simulink model "multilevelinverterc"  (R2014b)
settings: Solver=ode45  StartTime=0.0  StopTime=0.1  MaxStep=.00001  RelTol=1e-3
libraries: powerlib x58, simulink x10
settings Model: Creator=Muruganandham  LastModifiedBy=SELVA
settings DataIOCC: SignalLoggingSaveFormat=ModelDataLogs
settings OptimizationCC: ExpressionDepthLimit=2147483647
settings DebuggingCC: UnderspecifiedInitializationDetection=Classic  MergeDetectMultiDrivingBlocksExec=none  FcnCallInpInsideContextMsg=UseLocalSettings  StateNameClashWarn=warning
settings GRTTargetCC: CombineOutputUpdateFcns=off  GRTInterface=on

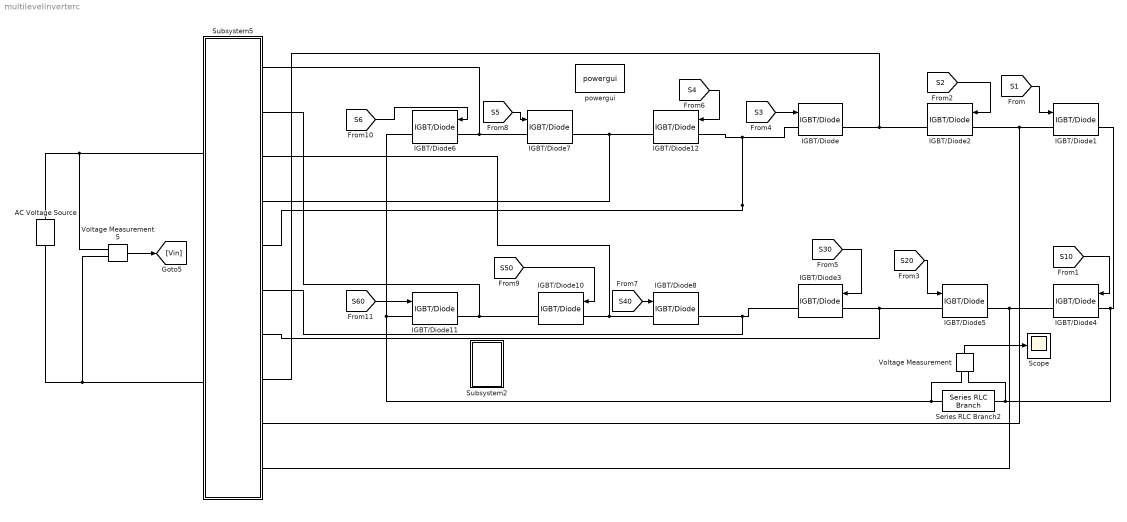
== system multilevelinverterc ==
  AC Voltage Source : powerlib/Electrical Sources/AC Voltage Source  Amplitude=230*sqrt(2)  Phase=0  Frequency=50  SampleTime=0  Measurements=None
  IGBT/Diode{,1..8,10..12} (12 alike) : powerlib/Power Electronics/IGBT//Diode  Ron=1e-3  Rs=1e5  Cs=inf  Measurements=on
  Scope : Scope
      settings: YMin=-600  YMax=600  SaveName=bh
  Series RLC Branch2 : powerlib/Elements/Series RLC Branch  LConnTagsString=__new0  RConnTagsString=__new0  BranchType=R  Resistance=10  Inductance=1e-3  SetiL0=off  InitialCurrent=0  Capacitance=1e-6  Setx0=off  InitialVoltage=0  Measurements=None
  Subsystem2 : Subsystem  mask{fc=10000, m=1}
      mask prompts: fc "Switching frequency"; m "modulation index"
  Subsystem5 : Subsystem
  Voltage Measurement : powerlib/Measurements/Voltage Measurement  PhasorSimulation=off  OutputType=Complex  PSBequivalent=0
  Voltage Measurement5 : powerlib/Measurements/Voltage Measurement  PhasorSimulation=off  OutputType=Complex  PSBequivalent=0
  powergui : powerlib/powergui  Priority=1  SimulationMode=Discrete  SolverType=Tustin  SampleTime=50e-6  frequency=60  SPID=off  DisableSnubberDevices=off  DisableRonSwitches=off  DisableVfSwitches=off  SwTol=0  DisplayEquations=off  Interpol=off  methode=off  Ts=0  frequencyindice=0  Pbase=100e6  ErrMax=1e-4  Iterations=50  UnitsV=kV  UnitsW=MW  FunctionMessages=off  echomessages=off  HookPort=off  EnableUseOfTLC=off  x0status=blocks  RestoreLinks=warning  ResistiveCurrentMeasurement=off  Frange=[0:2:500]  Ylog=off  Xlog=on  ShowGrid=off  save=off  variable=ZData  structure=bh  ZoomFFT=off  StartTime=0.04  cycles=1  DisplayStyle=1  fundamental=50  FreqAxis=off  MaxFrequency=10000  frequencyindicesteady=1  RmsSteady=1  display=off
  wires:
  [S1] -> IGBT/Diode1/1
  [S10] -> IGBT/Diode4/1
  [S2] -> IGBT/Diode2/1
  [S20] -> IGBT/Diode5/1
  [S3] -> IGBT/Diode/1
  [S30] -> IGBT/Diode3/1
  Voltage Measurement/1 -> Scope/1
  [S40] -> IGBT/Diode8/1
  [S6] -> IGBT/Diode6/1
  [S4] -> IGBT/Diode12/1
  [S5] -> IGBT/Diode7/1
  [S50] -> IGBT/Diode10/1
  [S60] -> IGBT/Diode11/1
  Voltage Measurement5/1 -> [Vin]
  connections:
  IGBT/Diode/RConn1 -- Subsystem5/RConn8 -- IGBT/Diode2/RConn1
  IGBT/Diode1/LConn1 -- IGBT/Diode2/LConn1 -- Subsystem5/RConn9
  IGBT/Diode3/LConn1 -- Subsystem5/RConn7 -- IGBT/Diode5/LConn1
  IGBT/Diode5/RConn1 -- Subsystem5/RConn10 -- IGBT/Diode4/RConn1
  IGBT/Diode1/RConn1 -- Voltage Measurement/LConn2 -- Series RLC Branch2/RConn1 -- IGBT/Diode4/LConn1
  IGBT/Diode6/LConn1 -- Subsystem5/RConn1 -- IGBT/Diode7/LConn1
  IGBT/Diode7/RConn1 -- Subsystem5/RConn4 -- IGBT/Diode12/RConn1
  IGBT/Diode11/RConn1 -- Subsystem5/RConn2 -- IGBT/Diode10/RConn1
  IGBT/Diode10/LConn1 -- Subsystem5/RConn3 -- IGBT/Diode8/LConn1
  IGBT/Diode/LConn1 -- Subsystem5/RConn5 -- IGBT/Diode12/LConn1
  IGBT/Diode3/RConn1 -- Subsystem5/RConn6 -- IGBT/Diode8/RConn1
  Series RLC Branch2/LConn1 -- IGBT/Diode11/LConn1 -- IGBT/Diode6/RConn1 -- Voltage Measurement/LConn1
  Voltage Measurement5/LConn1 -- AC Voltage Source/RConn1 -- Subsystem5/LConn1
  Voltage Measurement5/LConn2 -- AC Voltage Source/LConn1 -- Subsystem5/LConn2

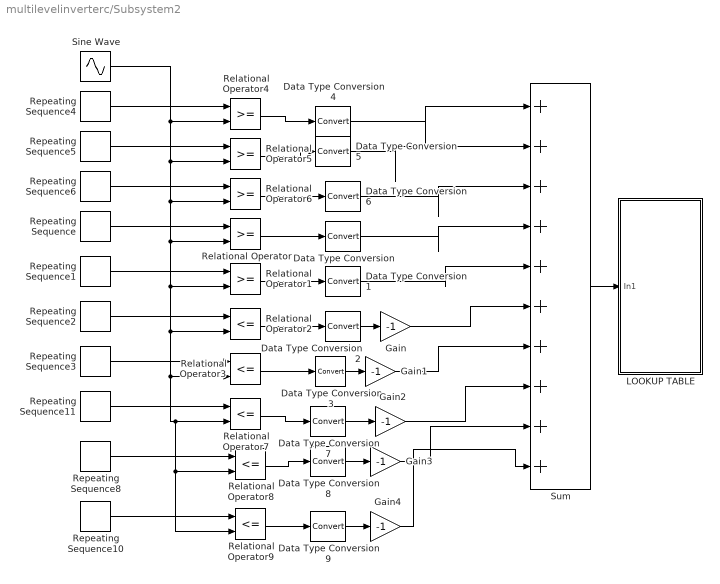
== system multilevelinverterc/Subsystem2 ==
  Data Type Conversion{,1..9} (10 alike) : DataTypeConversion
  Gain{,1..4} (5 alike) : Gain  Gain=-1
  LOOKUP TABLE : Subsystem
  Relational Operator{,1,4..6} (5 alike) : RelationalOperator  OutDataTypeStr=boolean
  Relational Operator{2..3,7..9} (5 alike) : RelationalOperator  Operator=<=  OutDataTypeStr=boolean
  Repeating Sequence : simulink/Sources/Repeating Sequence  rep_seq_t="[0 (1/fc)/2  (1/fc)]"  rep_seq_y=[2 1 2]
  Repeating Sequence1 : simulink/Sources/Repeating Sequence  rep_seq_t="[0 (1/fc)/2  (1/fc)]"  rep_seq_y=[1 0 1]
  Repeating Sequence10 : simulink/Sources/Repeating Sequence  rep_seq_t="[0 (1/fc)/2  (1/fc)]"  rep_seq_y=[-5 -4 -5]
  Repeating Sequence11 : simulink/Sources/Repeating Sequence  rep_seq_t="[0 (1/fc)/2  (1/fc)]"  rep_seq_y=[-3 -2 -3]
  Repeating Sequence2 : simulink/Sources/Repeating Sequence  rep_seq_t="[0 (1/fc)/2  (1/fc)]"  rep_seq_y=[-1 0 -1]
  Repeating Sequence3 : simulink/Sources/Repeating Sequence  rep_seq_t="[0 (1/fc)/2  (1/fc)]"  rep_seq_y=[-2 -1 -2]
  Repeating Sequence4 : simulink/Sources/Repeating Sequence  rep_seq_t="[0 (1/fc)/2  (1/fc)]"  rep_seq_y=[4 5 4]
  Repeating Sequence5 : simulink/Sources/Repeating Sequence  rep_seq_t="[0 (1/fc)/2  (1/fc)]"  rep_seq_y=[4 3 4]
  Repeating Sequence6 : simulink/Sources/Repeating Sequence  rep_seq_t="[0 (1/fc)/2  (1/fc)]"  rep_seq_y=[3 2 3]
  Repeating Sequence8 : simulink/Sources/Repeating Sequence  rep_seq_t="[0 (1/fc)/2  (1/fc)]"  rep_seq_y=[-4 -3 -4]
  Sine Wave : Sin  Amplitude=5*m  Frequency=2*pi*50  SampleTime=0
  Sum : Sum  Inputs=|++++++++++
  wires:
  Data Type Conversion3/1 -> Gain1/1
  Data Type Conversion2/1 -> Gain/1
  Relational Operator3/1 -> Data Type Conversion3/1
  Relational Operator2/1 -> Data Type Conversion2/1
  Repeating Sequence3/1 -> Relational Operator3/1
  Repeating Sequence2/1 -> Relational Operator2/1
  Repeating Sequence1/1 -> Relational Operator1/1
  Repeating Sequence/1 -> Relational Operator/1
  Relational Operator1/1 -> Data Type Conversion1/1
  Relational Operator/1 -> Data Type Conversion/1
  Repeating Sequence6/1 -> Relational Operator6/1
  Repeating Sequence5/1 -> Relational Operator5/1
  Repeating Sequence4/1 -> Relational Operator4/1
  Relational Operator6/1 -> Data Type Conversion6/1
  Relational Operator5/1 -> Data Type Conversion5/1
  Relational Operator4/1 -> Data Type Conversion4/1
  Repeating Sequence8/1 -> Relational Operator8/1
  Repeating Sequence11/1 -> Relational Operator7/1
  Relational Operator9/1 -> Data Type Conversion9/1
  Relational Operator8/1 -> Data Type Conversion8/1
  Relational Operator7/1 -> Data Type Conversion7/1
  Data Type Conversion9/1 -> Gain4/1
  Data Type Conversion8/1 -> Gain3/1
  Data Type Conversion7/1 -> Gain2/1
  Repeating Sequence10/1 -> Relational Operator9/1
  Data Type Conversion4/1 -> Sum/1
  Data Type Conversion5/1 -> Sum/2
  Data Type Conversion6/1 -> Sum/3
  Data Type Conversion/1 -> Sum/4
  Data Type Conversion1/1 -> Sum/5
  Gain/1 -> Sum/6
  Gain1/1 -> Sum/7
  Gain2/1 -> Sum/8
  Gain3/1 -> Sum/9
  Gain4/1 -> Sum/10
  Sum/1 -> LOOKUP TABLE/1(In1)
  Sine Wave/1 -> Relational Operator5/2, Relational Operator6/2, Relational Operator/2, Relational Operator1/2, Relational Operator2/2, Relational Operator3/2, Relational Operator7/2, Relational Operator9/2, Relational Operator8/2, Relational Operator4/2

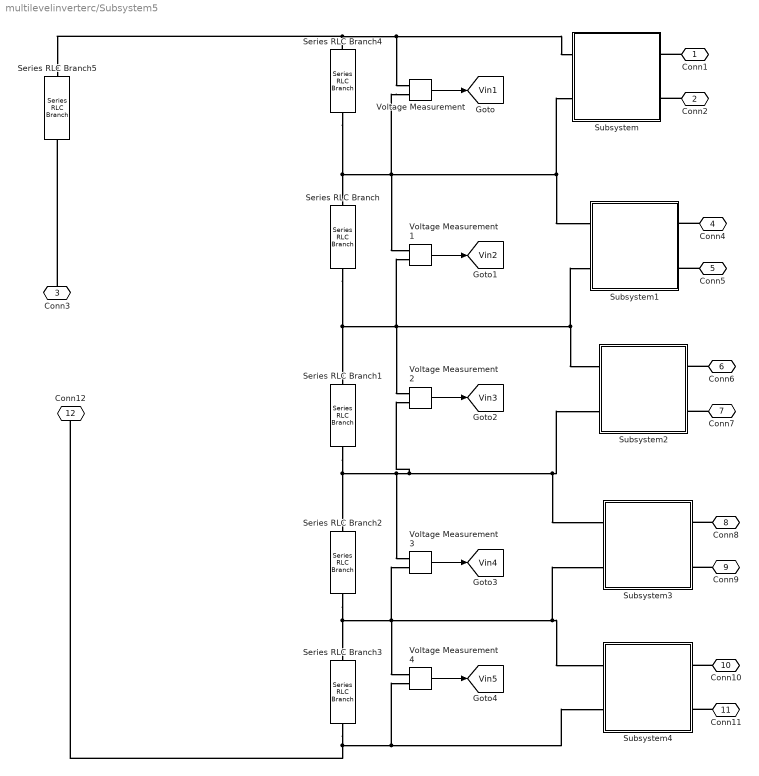
== system multilevelinverterc/Subsystem5 ==
  Series RLC Branch{,1..4} (5 alike) : powerlib/Elements/Series RLC Branch  LConnTagsString=__new0  RConnTagsString=__new0  BranchType=C  Resistance=1  Inductance=1e-3  SetiL0=off  InitialCurrent=0  Capacitance=2500e-6  Setx0=off  InitialVoltage=0  Measurements=None
  Series RLC Branch5 : powerlib/Elements/Series RLC Branch  LConnTagsString=__new0  RConnTagsString=__new0  BranchType=R  Resistance=.001  Inductance=1e-3  SetiL0=off  InitialCurrent=0  Capacitance=2500e-6  Setx0=off  InitialVoltage=0  Measurements=None
  Subsystem : Subsystem
  Subsystem1 : Subsystem
  Subsystem2 : Subsystem
  Subsystem3 : Subsystem
  Subsystem4 : Subsystem
  Voltage Measurement{,1..4} (5 alike) : powerlib/Measurements/Voltage Measurement  PhasorSimulation=off  OutputType=Complex  PSBequivalent=0
  Conn1 : PMIOPort  Port=1  Side=Right
  Conn2 : PMIOPort  Port=2  Side=Right
  Conn3 : PMIOPort  Port=3  Side=Left
  Conn4 : PMIOPort  Port=4  Side=Right
  Conn5 : PMIOPort  Port=5  Side=Right
  Conn6 : PMIOPort  Port=6  Side=Right
  Conn7 : PMIOPort  Port=7  Side=Right
  Conn8 : PMIOPort  Port=8  Side=Right
  Conn9 : PMIOPort  Port=9  Side=Right
  Conn10 : PMIOPort  Port=10  Side=Right
  Conn11 : PMIOPort  Port=11  Side=Right
  Conn12 : PMIOPort  Port=12  Side=Left
  tag scope: Vin1=global, Vin2=global, Vin3=global, Vin4=global, Vin5=global
  wires:
  Voltage Measurement/1 -> [Vin1]
  Voltage Measurement1/1 -> [Vin2]
  Voltage Measurement2/1 -> [Vin3]
  Voltage Measurement3/1 -> [Vin4]
  Voltage Measurement4/1 -> [Vin5]
  connections:
  Voltage Measurement/LConn2 -- Series RLC Branch4/RConn1 -- Series RLC Branch/LConn1 -- Subsystem/LConn2 -- Subsystem1/LConn1 -- Voltage Measurement1/LConn1
  Voltage Measurement1/LConn2 -- Series RLC Branch/RConn1 -- Series RLC Branch1/LConn1 -- Subsystem1/LConn2 -- Subsystem2/LConn1 -- Voltage Measurement2/LConn1
  Series RLC Branch1/RConn1 -- Subsystem2/LConn2 -- Subsystem3/LConn1 -- Voltage Measurement2/LConn2 -- Voltage Measurement3/LConn1 -- Series RLC Branch2/LConn1
  Series RLC Branch2/RConn1 -- Series RLC Branch3/LConn1 -- Subsystem3/LConn2 -- Subsystem4/LConn1 -- Voltage Measurement3/LConn2 -- Voltage Measurement4/LConn1
  Series RLC Branch3/RConn1 -- Conn12/RConn1 -- Subsystem4/LConn2 -- Voltage Measurement4/LConn2
  Series RLC Branch4/LConn1 -- Subsystem/LConn1 -- Voltage Measurement/LConn1 -- Series RLC Branch5/LConn1
  Conn1/RConn1 -- Subsystem/RConn1
  Conn2/RConn1 -- Subsystem/RConn2
  Conn3/RConn1 -- Series RLC Branch5/RConn1
  Conn4/RConn1 -- Subsystem1/RConn1
  Conn5/RConn1 -- Subsystem1/RConn2
  Conn6/RConn1 -- Subsystem2/RConn1
  Conn7/RConn1 -- Subsystem2/RConn2
  Conn8/RConn1 -- Subsystem3/RConn1
  Conn9/RConn1 -- Subsystem3/RConn2
  Conn10/RConn1 -- Subsystem4/RConn1
  Conn11/RConn1 -- Subsystem4/RConn2

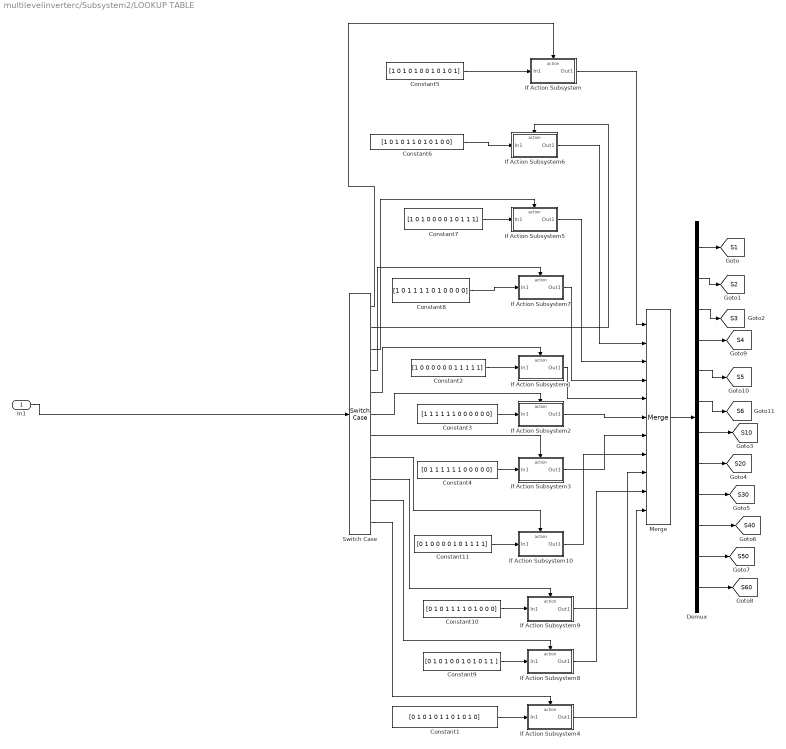
== system multilevelinverterc/Subsystem2/LOOKUP TABLE ==
  In1 : Inport
  Constant1 : Constant  Value=[0 1 0 1 0 1 1 0 1 0 1 0]
  Constant10 : Constant  Value=[0 1 0 1 1 1 1 0 1 0 0 0]
  Constant11 : Constant  Value=[0 1 0 0 0 0 1 0 1 1 1 1]
  Constant2 : Constant  Value=[1 0 0 0 0 0 0 1 1 1 1 1]
  Constant3 : Constant  Value=[1 1 1 1 1 1 0 0 0 0 0 0]
  Constant4 : Constant  Value=[0 1 1 1 1 1 1 0 0 0 0 0]
  Constant5 : Constant  Value=[1 0 1 0 1 0 0 1 0 1 0 1]
  Constant6 : Constant  Value=[1 0 1 0 1 1 0 1 0 1 0 0]
  Constant7 : Constant  Value=[1 0 1 0 0 0 0 1 0 1 1 1]
  Constant8 : Constant  Value=[1 0 1 1 1 1 0 1 0 0 0 0]
  Constant9 : Constant  Value=[0 1 0 1 0 0 1 0 1 0 1 1 ]
  Demux : Demux  Outputs=12
  If Action Subsystem : Subsystem  TreatAsAtomicUnit=on
  If Action Subsystem1 : Subsystem  TreatAsAtomicUnit=on
  If Action Subsystem10 : Subsystem  TreatAsAtomicUnit=on
  If Action Subsystem2 : Subsystem  TreatAsAtomicUnit=on
  If Action Subsystem3 : Subsystem  TreatAsAtomicUnit=on
  If Action Subsystem4 : Subsystem  TreatAsAtomicUnit=on
  If Action Subsystem5 : Subsystem  TreatAsAtomicUnit=on
  If Action Subsystem6 : Subsystem  TreatAsAtomicUnit=on
  If Action Subsystem7 : Subsystem  TreatAsAtomicUnit=on
  If Action Subsystem8 : Subsystem  TreatAsAtomicUnit=on
  If Action Subsystem9 : Subsystem  TreatAsAtomicUnit=on
  Merge : Merge  Inputs=11
  Switch Case : SwitchCase  CaseConditions={-5 -4 -3 -2 -1 0 1 2 3 4 5}  ShowDefaultCase=off
  tag scope: S10=global, S1=global, S20=global, S2=global, S30=global, S3=global, S40=global, S4=global, S50=global, S5=global, S60=global, S6=global
  wires:
  Merge/1 -> Demux/1
  If Action Subsystem/1(Out1) -> Merge/1
  Constant4/1 -> If Action Subsystem3/1(In1)
  Constant3/1 -> If Action Subsystem2/1(In1)
  Constant2/1 -> If Action Subsystem1/1(In1)
  Switch Case/6 -> If Action Subsystem2/Action
  If Action Subsystem6/1(Out1) -> Merge/2
  If Action Subsystem5/1(Out1) -> Merge/3
  If Action Subsystem7/1(Out1) -> Merge/4
  If Action Subsystem1/1(Out1) -> Merge/5
  If Action Subsystem2/1(Out1) -> Merge/6
  If Action Subsystem3/1(Out1) -> Merge/7
  Constant9/1 -> If Action Subsystem8/1(In1)
  Constant10/1 -> If Action Subsystem9/1(In1)
  Constant11/1 -> If Action Subsystem10/1(In1)
  Switch Case/11 -> If Action Subsystem4/Action
  If Action Subsystem4/1(Out1) -> Merge/11
  Switch Case/10 -> If Action Subsystem8/Action
  Switch Case/9 -> If Action Subsystem9/Action
  Switch Case/8 -> If Action Subsystem10/Action
  Switch Case/7 -> If Action Subsystem3/Action
  Switch Case/5 -> If Action Subsystem1/Action
  Switch Case/4 -> If Action Subsystem7/Action
  Switch Case/3 -> If Action Subsystem5/Action
  Switch Case/2 -> If Action Subsystem6/Action
  Switch Case/1 -> If Action Subsystem/Action
  Constant6/1 -> If Action Subsystem6/1(In1)
  Constant7/1 -> If Action Subsystem5/1(In1)
  Constant8/1 -> If Action Subsystem7/1(In1)
  If Action Subsystem10/1(Out1) -> Merge/8
  If Action Subsystem9/1(Out1) -> Merge/9
  If Action Subsystem8/1(Out1) -> Merge/10
  Demux/3 -> [S3]
  Demux/2 -> [S2]
  Demux/1 -> [S1]
  Demux/7 -> [S10]
  Demux/8 -> [S20]
  Demux/9 -> [S30]
  Demux/10 -> [S40]
  Demux/11 -> [S50]
  Demux/12 -> [S60]
  Demux/6 -> [S6]
  Demux/5 -> [S5]
  Demux/4 -> [S4]
  Constant1/1 -> If Action Subsystem4/1(In1)
  Constant5/1 -> If Action Subsystem/1(In1)
  In1/1 -> Switch Case/1

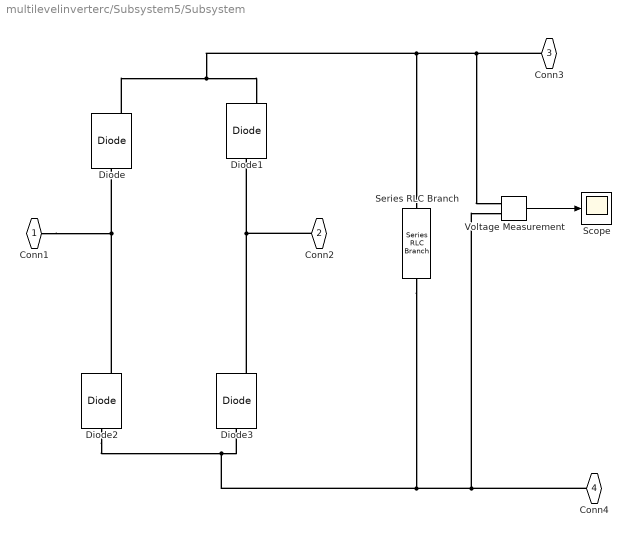
== system multilevelinverterc/Subsystem5/Subsystem ==
  Diode{,1..3} (4 alike) : powerlib/Power Electronics/Diode  Ron=0.001  Lon=0  Vf=0.8  IC=0  UseSnubber=off  Rs=500  Cs=250e-9  Measurements=on
  Scope : Scope
      settings: TimeRange=1.601532567049809  YMin=9.312500000000002  YMax=11.5625
  Series RLC Branch : powerlib/Elements/Series RLC Branch  LConnTagsString=__new0  RConnTagsString=__new0  BranchType=C  Resistance=1  Inductance=1e-3  SetiL0=off  InitialCurrent=0  Capacitance=25000e-6  Setx0=off  InitialVoltage=0  Measurements=None
  Voltage Measurement : powerlib/Measurements/Voltage Measurement  PhasorSimulation=off  OutputType=Complex  PSBequivalent=0
  Conn1 : PMIOPort  Port=1  Side=Left
  Conn2 : PMIOPort  Port=2  Side=Left
  Conn3 : PMIOPort  Port=3  Side=Right
  Conn4 : PMIOPort  Port=4  Side=Right
  wires:
  Voltage Measurement/1 -> Scope/1
  connections:
  Conn4/RConn1 -- Voltage Measurement/LConn2 -- Diode2/LConn1 -- Diode3/LConn1 -- Series RLC Branch/RConn1
  Diode2/RConn1 -- Diode/LConn1 -- Conn1/RConn1
  Conn3/RConn1 -- Voltage Measurement/LConn1 -- Diode/RConn1 -- Diode1/RConn1 -- Series RLC Branch/LConn1
  Diode3/RConn1 -- Diode1/LConn1 -- Conn2/RConn1

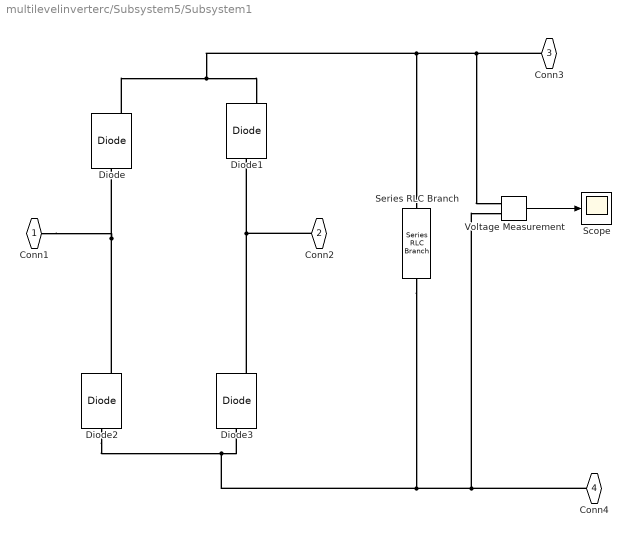
== system multilevelinverterc/Subsystem5/Subsystem1 ==
  Diode{,1..3} (4 alike) : powerlib/Power Electronics/Diode  Ron=0.001  Lon=0  Vf=0.8  IC=0  UseSnubber=off  Rs=500  Cs=250e-9  Measurements=on
  Scope : Scope
      settings: TimeRange=1.601532567049809  YMin=9.312500000000002  YMax=11.5625
  Series RLC Branch : powerlib/Elements/Series RLC Branch  LConnTagsString=__new0  RConnTagsString=__new0  BranchType=C  Resistance=1  Inductance=1e-3  SetiL0=off  InitialCurrent=0  Capacitance=25000e-6  Setx0=off  InitialVoltage=0  Measurements=None
  Voltage Measurement : powerlib/Measurements/Voltage Measurement  PhasorSimulation=off  OutputType=Complex  PSBequivalent=0
  Conn1 : PMIOPort  Port=1  Side=Left
  Conn2 : PMIOPort  Port=2  Side=Left
  Conn3 : PMIOPort  Port=3  Side=Right
  Conn4 : PMIOPort  Port=4  Side=Right
  wires:
  Voltage Measurement/1 -> Scope/1
  connections:
  Conn2/RConn1 -- Diode1/LConn1 -- Diode3/RConn1
  Conn3/RConn1 -- Series RLC Branch/LConn1 -- Diode1/RConn1 -- Diode/RConn1 -- Voltage Measurement/LConn1
  Conn1/RConn1 -- Diode/LConn1 -- Diode2/RConn1
  Conn4/RConn1 -- Series RLC Branch/RConn1 -- Diode3/LConn1 -- Diode2/LConn1 -- Voltage Measurement/LConn2

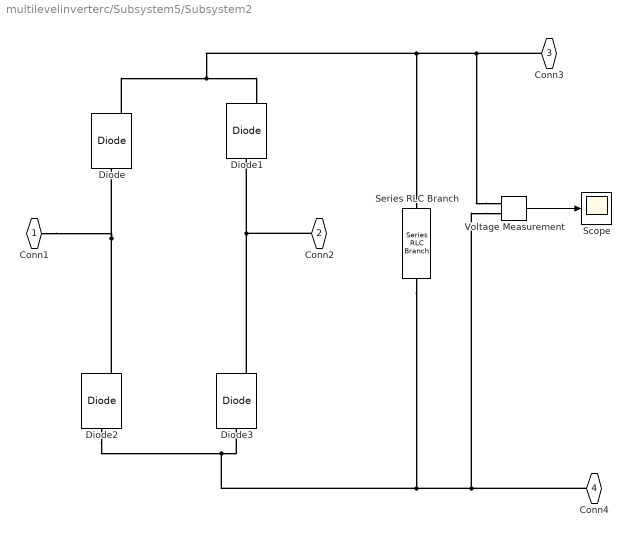
== system multilevelinverterc/Subsystem5/Subsystem2 ==
  Diode{,1..3} (4 alike) : powerlib/Power Electronics/Diode  Ron=0.001  Lon=0  Vf=0.8  IC=0  UseSnubber=off  Rs=500  Cs=250e-9  Measurements=on
  Scope : Scope
      settings: TimeRange=1.601532567049809  YMin=9.312500000000002  YMax=11.5625
  Series RLC Branch : powerlib/Elements/Series RLC Branch  LConnTagsString=__new0  RConnTagsString=__new0  BranchType=C  Resistance=1  Inductance=1e-3  SetiL0=off  InitialCurrent=0  Capacitance=25000e-6  Setx0=off  InitialVoltage=0  Measurements=None
  Voltage Measurement : powerlib/Measurements/Voltage Measurement  PhasorSimulation=off  OutputType=Complex  PSBequivalent=0
  Conn1 : PMIOPort  Port=1  Side=Left
  Conn2 : PMIOPort  Port=2  Side=Left
  Conn3 : PMIOPort  Port=3  Side=Right
  Conn4 : PMIOPort  Port=4  Side=Right
  wires:
  Voltage Measurement/1 -> Scope/1
  connections:
  Voltage Measurement/LConn2 -- Diode2/LConn1 -- Diode3/LConn1 -- Series RLC Branch/RConn1 -- Conn4/RConn1
  Diode2/RConn1 -- Diode/LConn1 -- Conn1/RConn1
  Voltage Measurement/LConn1 -- Diode/RConn1 -- Diode1/RConn1 -- Series RLC Branch/LConn1 -- Conn3/RConn1
  Diode3/RConn1 -- Diode1/LConn1 -- Conn2/RConn1

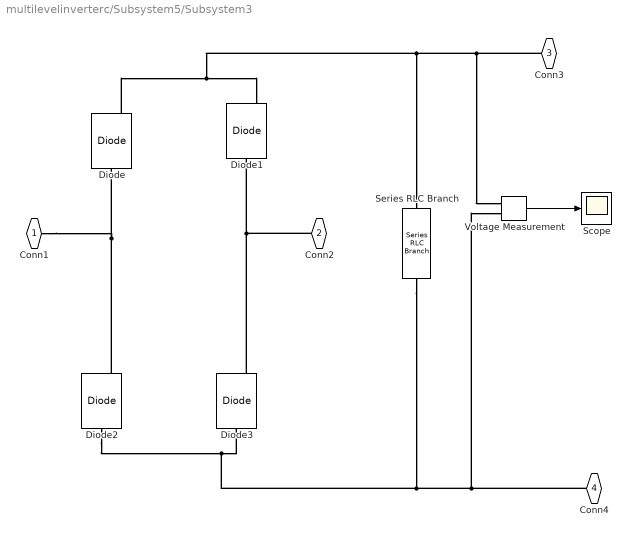
== system multilevelinverterc/Subsystem5/Subsystem3 ==
  Diode{,1..3} (4 alike) : powerlib/Power Electronics/Diode  Ron=0.001  Lon=0  Vf=0.8  IC=0  UseSnubber=off  Rs=500  Cs=250e-9  Measurements=on
  Scope : Scope
      settings: TimeRange=1.601532567049809  YMin=9.312500000000002  YMax=11.5625
  Series RLC Branch : powerlib/Elements/Series RLC Branch  LConnTagsString=__new0  RConnTagsString=__new0  BranchType=C  Resistance=1  Inductance=1e-3  SetiL0=off  InitialCurrent=0  Capacitance=25000e-6  Setx0=off  InitialVoltage=0  Measurements=None
  Voltage Measurement : powerlib/Measurements/Voltage Measurement  PhasorSimulation=off  OutputType=Complex  PSBequivalent=0
  Conn1 : PMIOPort  Port=1  Side=Left
  Conn2 : PMIOPort  Port=2  Side=Left
  Conn3 : PMIOPort  Port=3  Side=Right
  Conn4 : PMIOPort  Port=4  Side=Right
  wires:
  Voltage Measurement/1 -> Scope/1
  connections:
  Conn2/RConn1 -- Diode1/LConn1 -- Diode3/RConn1
  Conn3/RConn1 -- Series RLC Branch/LConn1 -- Diode1/RConn1 -- Diode/RConn1 -- Voltage Measurement/LConn1
  Conn1/RConn1 -- Diode/LConn1 -- Diode2/RConn1
  Conn4/RConn1 -- Series RLC Branch/RConn1 -- Diode3/LConn1 -- Diode2/LConn1 -- Voltage Measurement/LConn2

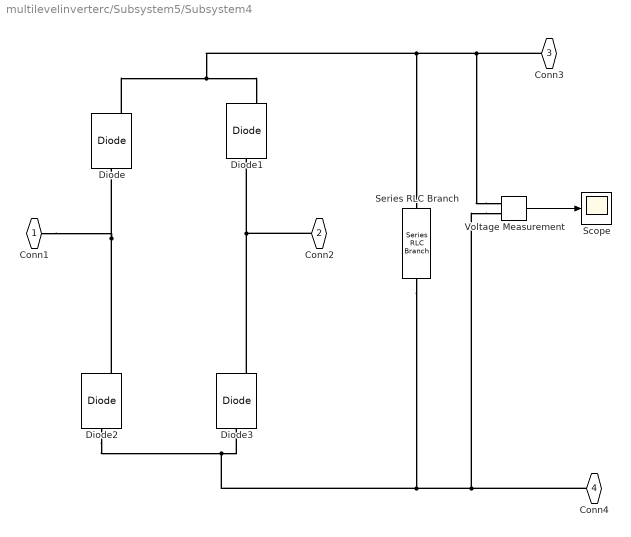
== system multilevelinverterc/Subsystem5/Subsystem4 ==
  Diode{,1..3} (4 alike) : powerlib/Power Electronics/Diode  Ron=0.001  Lon=0  Vf=0.8  IC=0  UseSnubber=off  Rs=500  Cs=250e-9  Measurements=on
  Scope : Scope
      settings: TimeRange=1.601532567049809  YMin=9.312500000000002  YMax=11.5625
  Series RLC Branch : powerlib/Elements/Series RLC Branch  LConnTagsString=__new0  RConnTagsString=__new0  BranchType=C  Resistance=1  Inductance=1e-3  SetiL0=off  InitialCurrent=0  Capacitance=25000e-6  Setx0=off  InitialVoltage=0  Measurements=None
  Voltage Measurement : powerlib/Measurements/Voltage Measurement  PhasorSimulation=off  OutputType=Complex  PSBequivalent=0
  Conn1 : PMIOPort  Port=1  Side=Left
  Conn2 : PMIOPort  Port=2  Side=Left
  Conn3 : PMIOPort  Port=3  Side=Right
  Conn4 : PMIOPort  Port=4  Side=Right
  wires:
  Voltage Measurement/1 -> Scope/1
  connections:
  Voltage Measurement/LConn2 -- Diode2/LConn1 -- Diode3/LConn1 -- Series RLC Branch/RConn1 -- Conn4/RConn1
  Diode2/RConn1 -- Diode/LConn1 -- Conn1/RConn1
  Voltage Measurement/LConn1 -- Diode/RConn1 -- Diode1/RConn1 -- Series RLC Branch/LConn1 -- Conn3/RConn1
  Diode3/RConn1 -- Diode1/LConn1 -- Conn2/RConn1

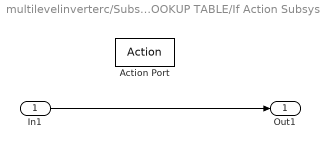
== system multilevelinverterc/Subsystem2/LOOKUP TABLE/If Action Subsystem ==
  In1 : Inport
  Action Port : ActionPort  ActionType=case
  Out1 : Outport
  wires:
  In1/1 -> Out1/1

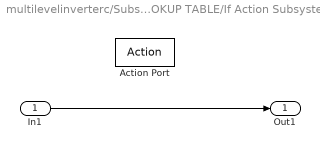
== system multilevelinverterc/Subsystem2/LOOKUP TABLE/If Action Subsystem1 ==
  In1 : Inport
  Action Port : ActionPort  ActionType=case
  Out1 : Outport
  wires:
  In1/1 -> Out1/1

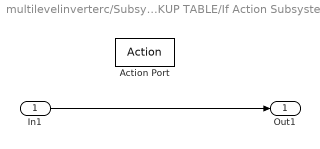
== system multilevelinverterc/Subsystem2/LOOKUP TABLE/If Action Subsystem10 ==
  In1 : Inport
  Action Port : ActionPort  ActionType=case
  Out1 : Outport
  wires:
  In1/1 -> Out1/1

== system multilevelinverterc/Subsystem2/LOOKUP TABLE/If Action Subsystem2 ==
  In1 : Inport
  Action Port : ActionPort  ActionType=case
  Out1 : Outport
  wires:
  In1/1 -> Out1/1

== system multilevelinverterc/Subsystem2/LOOKUP TABLE/If Action Subsystem3 ==
  In1 : Inport
  Action Port : ActionPort  ActionType=case
  Out1 : Outport
  wires:
  In1/1 -> Out1/1

== system multilevelinverterc/Subsystem2/LOOKUP TABLE/If Action Subsystem4 ==
  In1 : Inport
  Action Port : ActionPort  ActionType=case
  Out1 : Outport
  wires:
  In1/1 -> Out1/1

== system multilevelinverterc/Subsystem2/LOOKUP TABLE/If Action Subsystem5 ==
  In1 : Inport
  Action Port : ActionPort  ActionType=case
  Out1 : Outport
  wires:
  In1/1 -> Out1/1

== system multilevelinverterc/Subsystem2/LOOKUP TABLE/If Action Subsystem6 ==
  In1 : Inport
  Action Port : ActionPort  ActionType=case
  Out1 : Outport
  wires:
  In1/1 -> Out1/1

== system multilevelinverterc/Subsystem2/LOOKUP TABLE/If Action Subsystem7 ==
  In1 : Inport
  Action Port : ActionPort  ActionType=case
  Out1 : Outport
  wires:
  In1/1 -> Out1/1

== system multilevelinverterc/Subsystem2/LOOKUP TABLE/If Action Subsystem8 ==
  In1 : Inport
  Action Port : ActionPort  ActionType=case
  Out1 : Outport
  wires:
  In1/1 -> Out1/1

== system multilevelinverterc/Subsystem2/LOOKUP TABLE/If Action Subsystem9 ==
  In1 : Inport
  Action Port : ActionPort  ActionType=case
  Out1 : Outport
  wires:
  In1/1 -> Out1/1
